simulink library "peripheral_utilities_src"  (R2022b)
settings: Solver=VariableStepAuto  StartTime=0.0  StopTime=10.0  RelTol=1e-3
libraries: $bdroot x16, simulink x5, spsSeriesRLCBranchLib x3, peripheral_utilities x3, spsVoltageMeasurementLib x2, spsMosfetLib x2, spsCurrentMeasurementLib x1, spsSecondOrderFilterLib x1, spsGroundLib x1
(part 2 of 2)

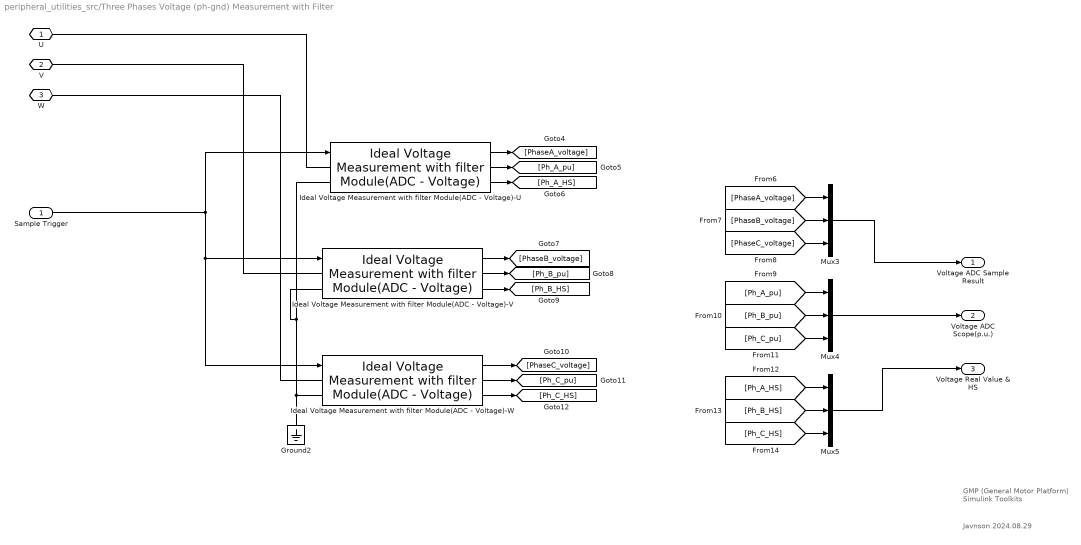
== system peripheral_utilities_src/Three Phases Voltage (ph-gnd) Measurement with Filter ==
  note: Javnson
      | 2024.08.29
  note: GMP (General Motor Platform)
      | Simulink Toolkits
  Sample Trigger : Inport
  Ground2 : spsGroundLib/Ground  LConnTagsString=a
  Ideal Voltage Measurement with filter Module(ADC - Voltage)-U : $bdroot/Ideal Voltage Measurement with filter Module(ADC - Voltage)  ADC_GAIN=ADC_GAIN  ADC_BIT=ADC_BIT  ADC_REFERENCE=ADC_REFERENCE  ADC_BIAS=ADC_BIAS  ADC_INIT=ADC_INIT  cut_frequency=cut_frequency
  Ideal Voltage Measurement with filter Module(ADC - Voltage)-V : $bdroot/Ideal Voltage Measurement with filter Module(ADC - Voltage)  ADC_GAIN=ADC_GAIN  ADC_BIT=ADC_BIT  ADC_REFERENCE=ADC_REFERENCE  ADC_BIAS=ADC_BIAS  ADC_INIT=ADC_INIT  cut_frequency=cut_frequency
  Ideal Voltage Measurement with filter Module(ADC - Voltage)-W : $bdroot/Ideal Voltage Measurement with filter Module(ADC - Voltage)  ADC_GAIN=ADC_GAIN  ADC_BIT=ADC_BIT  ADC_REFERENCE=ADC_REFERENCE  ADC_BIAS=ADC_BIAS  ADC_INIT=ADC_INIT  cut_frequency=cut_frequency
  Mux3 : Mux  Inputs=3
  Mux4 : Mux  Inputs=3
  Mux5 : Mux  Inputs=3
  U : PMIOPort  Side=Left
  V : PMIOPort  Port=2  Side=Left
  W : PMIOPort  Port=3  Side=Left
  Voltage ADC Sample Result : Outport
  Voltage ADC Scope(p.u.) : Outport  Port=2
  Voltage Real Value & HS : Outport  Port=3
  wires:
  Ideal Voltage Measurement with filter Module(ADC - Voltage)-W/3 -> [Ph_C_HS]
  Sample Trigger/1 -> Ideal Voltage Measurement with filter Module(ADC - Voltage)-U/1, Ideal Voltage Measurement with filter Module(ADC - Voltage)-W/1, Ideal Voltage Measurement with filter Module(ADC - Voltage)-V/1
  Ideal Voltage Measurement with filter Module(ADC - Voltage)-V/2 -> [Ph_B_pu]
  Ideal Voltage Measurement with filter Module(ADC - Voltage)-V/3 -> [Ph_B_HS]
  Mux4/1 -> Voltage ADC Scope(p.u.)/1
  [Ph_B_HS] -> Mux5/2
  Ideal Voltage Measurement with filter Module(ADC - Voltage)-W/1 -> [PhaseC_voltage]
  Ideal Voltage Measurement with filter Module(ADC - Voltage)-V/1 -> [PhaseB_voltage]
  Ideal Voltage Measurement with filter Module(ADC - Voltage)-U/1 -> [PhaseA_voltage]
  Ideal Voltage Measurement with filter Module(ADC - Voltage)-U/2 -> [Ph_A_pu]
  [Ph_B_pu] -> Mux4/2
  [PhaseB_voltage] -> Mux3/2
  Ideal Voltage Measurement with filter Module(ADC - Voltage)-U/3 -> [Ph_A_HS]
  Ideal Voltage Measurement with filter Module(ADC - Voltage)-W/2 -> [Ph_C_pu]
  [Ph_A_pu] -> Mux4/1
  [PhaseC_voltage] -> Mux3/3
  [PhaseA_voltage] -> Mux3/1
  [Ph_C_pu] -> Mux4/3
  [Ph_C_HS] -> Mux5/3
  Mux3/1 -> Voltage ADC Sample Result/1
  [Ph_A_HS] -> Mux5/1
  Mux5/1 -> Voltage Real Value & HS/1
  connections:
  Ground2/LConn1 -- Ideal Voltage Measurement with filter Module(ADC - Voltage)-V/LConn2 -- Ideal Voltage Measurement with filter Module(ADC - Voltage)-U/LConn2 -- Ideal Voltage Measurement with filter Module(ADC - Voltage)-W/LConn2
  Ideal Voltage Measurement with filter Module(ADC - Voltage)-U/LConn1 -- U/RConn1
  Ideal Voltage Measurement with filter Module(ADC - Voltage)-V/LConn1 -- V/RConn1
  Ideal Voltage Measurement with filter Module(ADC - Voltage)-W/LConn1 -- W/RConn1

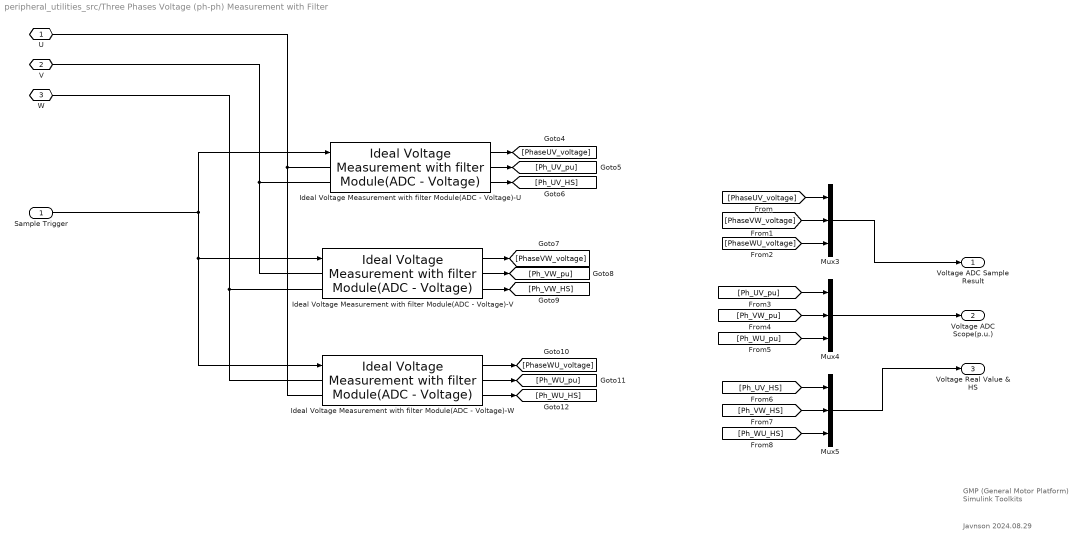
== system peripheral_utilities_src/Three Phases Voltage (ph-ph) Measurement with Filter ==
  note: Javnson
      | 2024.08.29
  note: GMP (General Motor Platform)
      | Simulink Toolkits
  Sample Trigger : Inport
  Ideal Voltage Measurement with filter Module(ADC - Voltage)-U : peripheral_utilities/Ideal Voltage Measurement with filter Module(ADC - Voltage)  ADC_GAIN=ADC_GAIN  ADC_BIT=ADC_BIT  ADC_REFERENCE=ADC_REFERENCE  ADC_BIAS=ADC_BIAS  ADC_INIT=ADC_INIT  cut_frequency=cut_frequency
  Ideal Voltage Measurement with filter Module(ADC - Voltage)-V : peripheral_utilities/Ideal Voltage Measurement with filter Module(ADC - Voltage)  ADC_GAIN=ADC_GAIN  ADC_BIT=ADC_BIT  ADC_REFERENCE=ADC_REFERENCE  ADC_BIAS=ADC_BIAS  ADC_INIT=ADC_INIT  cut_frequency=cut_frequency
  Ideal Voltage Measurement with filter Module(ADC - Voltage)-W : peripheral_utilities/Ideal Voltage Measurement with filter Module(ADC - Voltage)  ADC_GAIN=ADC_GAIN  ADC_BIT=ADC_BIT  ADC_REFERENCE=ADC_REFERENCE  ADC_BIAS=ADC_BIAS  ADC_INIT=ADC_INIT  cut_frequency=cut_frequency
  Mux3 : Mux  Inputs=3
  Mux4 : Mux  Inputs=3
  Mux5 : Mux  Inputs=3
  U : PMIOPort  Side=Left
  V : PMIOPort  Port=2  Side=Left
  W : PMIOPort  Port=3  Side=Left
  Voltage ADC Sample Result : Outport
  Voltage ADC Scope(p.u.) : Outport  Port=2
  Voltage Real Value & HS : Outport  Port=3
  wires:
  Ideal Voltage Measurement with filter Module(ADC - Voltage)-W/3 -> [Ph_WU_HS]
  Sample Trigger/1 -> Ideal Voltage Measurement with filter Module(ADC - Voltage)-U/1, Ideal Voltage Measurement with filter Module(ADC - Voltage)-V/1, Ideal Voltage Measurement with filter Module(ADC - Voltage)-W/1
  Ideal Voltage Measurement with filter Module(ADC - Voltage)-V/2 -> [Ph_VW_pu]
  Ideal Voltage Measurement with filter Module(ADC - Voltage)-V/3 -> [Ph_VW_HS]
  Mux4/1 -> Voltage ADC Scope(p.u.)/1
  [Ph_VW_HS] -> Mux5/2
  Ideal Voltage Measurement with filter Module(ADC - Voltage)-W/1 -> [PhaseWU_voltage]
  Ideal Voltage Measurement with filter Module(ADC - Voltage)-V/1 -> [PhaseVW_voltage]
  Ideal Voltage Measurement with filter Module(ADC - Voltage)-U/1 -> [PhaseUV_voltage]
  Ideal Voltage Measurement with filter Module(ADC - Voltage)-U/2 -> [Ph_UV_pu]
  [Ph_VW_pu] -> Mux4/2
  [PhaseVW_voltage] -> Mux3/2
  Ideal Voltage Measurement with filter Module(ADC - Voltage)-U/3 -> [Ph_UV_HS]
  Ideal Voltage Measurement with filter Module(ADC - Voltage)-W/2 -> [Ph_WU_pu]
  [Ph_UV_pu] -> Mux4/1
  [PhaseWU_voltage] -> Mux3/3
  [PhaseUV_voltage] -> Mux3/1
  [Ph_WU_pu] -> Mux4/3
  [Ph_WU_HS] -> Mux5/3
  Mux3/1 -> Voltage ADC Sample Result/1
  [Ph_UV_HS] -> Mux5/1
  Mux5/1 -> Voltage Real Value & HS/1
  connections:
  Ideal Voltage Measurement with filter Module(ADC - Voltage)-U/LConn1 -- Ideal Voltage Measurement with filter Module(ADC - Voltage)-W/LConn2 -- U/RConn1
  Ideal Voltage Measurement with filter Module(ADC - Voltage)-V/LConn1 -- Ideal Voltage Measurement with filter Module(ADC - Voltage)-U/LConn2 -- V/RConn1
  Ideal Voltage Measurement with filter Module(ADC - Voltage)-W/LConn1 -- Ideal Voltage Measurement with filter Module(ADC - Voltage)-V/LConn2 -- W/RConn1

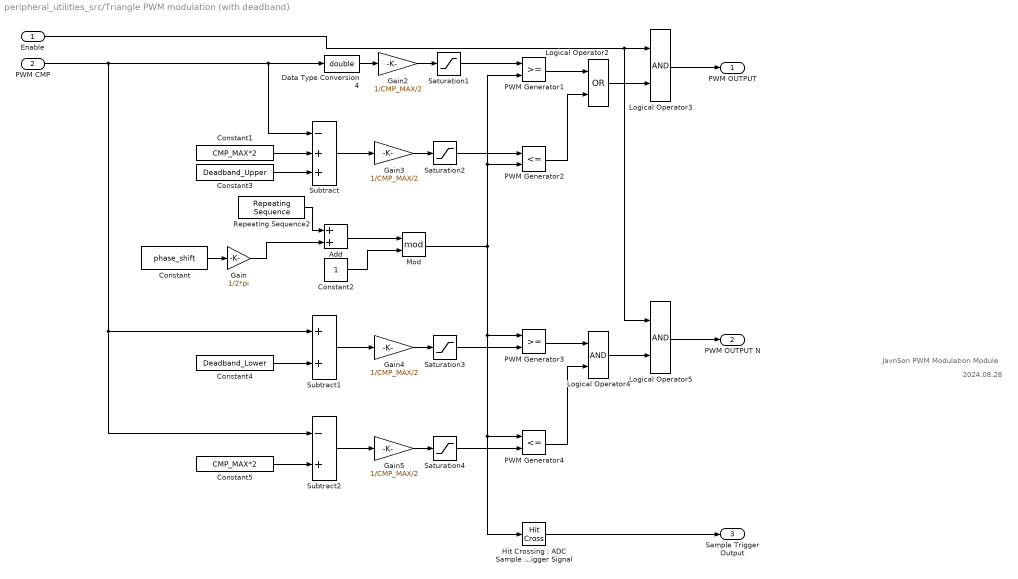
== system peripheral_utilities_src/Triangle PWM modulation (with deadband) ==
  note: 2024.08.28
  note: JavnSon PWM Modulation Module
  Enable : Inport
  PWM CMP : Inport  Port=2
  Add : Sum
  Constant : Constant  Value=phase_shift
  Constant1 : Constant  Value=CMP_MAX*2
  Constant2 : Constant
  Constant3 : Constant  Value=Deadband_Upper
  Constant4 : Constant  Value=Deadband_Lower
  Constant5 : Constant  Value=CMP_MAX*2
  Data Type Conversion4 : DataTypeConversion  OutDataTypeStr=double  SaturateOnIntegerOverflow=off  RndMeth=Floor
  Gain : Gain  Gain=1/2*pi
  Gain{2..5} (4 alike) : Gain  Gain=1/CMP_MAX/2
  Hit Crossing：ADC Sample Trigger Signal : HitCross  HitCrossingOffset=0.5  HitCrossingDirection=rising
  Logical Operator2 : Logic  Operator=OR  AllPortsSameDT=off  OutDataTypeStr=boolean
  Logical Operator3 : Logic  AllPortsSameDT=off  OutDataTypeStr=boolean
  Logical Operator4 : Logic  AllPortsSameDT=off  OutDataTypeStr=boolean
  Logical Operator5 : Logic  AllPortsSameDT=off  OutDataTypeStr=boolean
  Mod : Math  Operator=mod
  PWM Generator1 : RelationalOperator  OutDataTypeStr=boolean  InputSameDT=off
  PWM Generator2 : RelationalOperator  Operator=<=  OutDataTypeStr=boolean  InputSameDT=off
  PWM Generator3 : RelationalOperator  OutDataTypeStr=boolean  InputSameDT=off
  PWM Generator4 : RelationalOperator  Operator=<=  OutDataTypeStr=boolean  InputSameDT=off
  Repeating Sequence2 : simulink/Sources/Repeating Sequence  rep_seq_t=[0, 1/2/fswitch, 1/fswitch ]  rep_seq_y=[0,0.5,1]
  Saturation{1..4} (4 alike) : Saturate  UpperLimit=1  LowerLimit=0
  Subtract : Sum  Inputs=-++
  Subtract1 : Sum
  Subtract2 : Sum  Inputs=-+
  PWM OUTPUT : Outport
  PWM OUTPUT N : Outport  Port=2
  Sample Trigger Output : Outport  Port=3
  wires:
  PWM CMP/1 -> Subtract2/1, Subtract1/1, Subtract/1, Data Type Conversion4/1
  Data Type Conversion4/1 -> Gain2/1
  Gain2/1 -> Saturation1/1
  Saturation1/1 -> PWM Generator1/1
  PWM Generator1/1 -> Logical Operator2/1
  Logical Operator2/1 -> Logical Operator3/2
  Constant1/1 -> Subtract/2
  Constant3/1 -> Subtract/3
  PWM Generator2/1 -> Logical Operator2/2
  Gain3/1 -> Saturation2/1
  Subtract/1 -> Gain3/1
  Saturation2/1 -> PWM Generator2/1
  Constant4/1 -> Subtract1/2
  Gain4/1 -> Saturation3/1
  Subtract1/1 -> Gain4/1
  Saturation3/1 -> PWM Generator3/2
  PWM Generator3/1 -> Logical Operator4/1
  Constant5/1 -> Subtract2/2
  Saturation4/1 -> PWM Generator4/2
  Gain5/1 -> Saturation4/1
  Subtract2/1 -> Gain5/1
  PWM Generator4/1 -> Logical Operator4/2
  Logical Operator4/1 -> Logical Operator5/2
  Mod/1 -> PWM Generator2/2, PWM Generator1/2, PWM Generator3/1, Hit Crossing：ADC Sample Trigger Signal/1, PWM Generator4/1
  Enable/1 -> Logical Operator5/1, Logical Operator3/1
  Logical Operator5/1 -> PWM OUTPUT N/1
  Logical Operator3/1 -> PWM OUTPUT/1
  Hit Crossing：ADC Sample Trigger Signal/1 -> Sample Trigger Output/1
  Repeating Sequence2/1 -> Add/1
  Gain/1 -> Add/2
  Add/1 -> Mod/1
  Constant2/1 -> Mod/2
  Constant/1 -> Gain/1

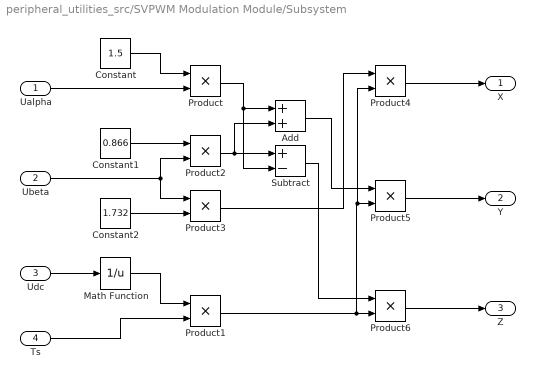
== system peripheral_utilities_src/SVPWM Modulation Module/Subsystem ==
  Ualpha : Inport
  Ubeta : Inport  Port=2
  Udc : Inport  Port=3
  Ts : Inport  Port=4
  Add : Sum
  Constant : Constant  Value=1.5
  Constant1 : Constant  Value=0.866
  Constant2 : Constant  Value=1.732
  Math Function : Math  Operator=reciprocal
  Product{,1..6} (7 alike) : Product
  Subtract : Sum  Inputs=+-
  X : Outport
  Y : Outport  Port=2
  Z : Outport  Port=3
  wires:
  Product1/1 -> Product4/2, Product5/2, Product6/2
  Ts/1 -> Product1/2
  Product6/1 -> Z/1
  Add/1 -> Product5/1
  Ualpha/1 -> Product/2
  Math Function/1 -> Product1/1
  Product2/1 -> Subtract/1, Add/2
  Product4/1 -> X/1
  Product3/1 -> Product4/1
  Constant/1 -> Product/1
  Constant1/1 -> Product2/1
  Ubeta/1 -> Product3/1, Product2/2
  Product5/1 -> Y/1
  Product/1 -> Add/1, Subtract/2
  Constant2/1 -> Product3/2
  Udc/1 -> Math Function/1
  Subtract/1 -> Product6/1

== system peripheral_utilities_src/SVPWM Modulation Module/Subsystem1 ==
  N : Inport
  X : Inport  Port=2
  Y : Inport  Port=3
  Z : Inport  Port=4
  Gain : Gain  Gain=-1
  Gain1 : Gain  Gain=-1
  Gain2 : Gain  Gain=-1
  Multiport Switch : MultiPortSwitch  Inputs=6  DiagnosticForDefault=None  SaturateOnIntegerOverflow=off  InputSameDT=off
  Multiport Switch1 : MultiPortSwitch  Inputs=6  DiagnosticForDefault=None  SaturateOnIntegerOverflow=off  InputSameDT=off
  T1 : Outport
  T2 : Outport  Port=2
  wires:
  Multiport Switch1/1 -> T2/1
  X/1 -> Multiport Switch1/4, Multiport Switch/6, Gain/1
  Y/1 -> Gain1/1, Multiport Switch/3, Multiport Switch1/2
  Z/1 -> Gain2/1, Multiport Switch/2, Multiport Switch1/5
  Gain/1 -> Multiport Switch1/3, Multiport Switch/5
  Gain2/1 -> Multiport Switch/4, Multiport Switch1/7
  N/1 -> Multiport Switch1/1, Multiport Switch/1
  Gain1/1 -> Multiport Switch1/6, Multiport Switch/7
  Multiport Switch/1 -> T1/1

== system peripheral_utilities_src/SVPWM Modulation Module/Subsystem2 ==
  N : Inport
  T1 : Inport  Port=2  Interpolate=off
  T2 : Inport  Port=3
  Ts : Inport  Port=4
  Add : Sum
  Add1 : Sum
  Constant : Constant  Value=0.25
  Constant1 : Constant  Value=0.5
  Constant2 : Constant  Value=0.5
  Multiport Switch : MultiPortSwitch  Inputs=6  DiagnosticForDefault=None  SaturateOnIntegerOverflow=off  InputSameDT=off
  Multiport Switch1 : MultiPortSwitch  Inputs=6  DiagnosticForDefault=None  SaturateOnIntegerOverflow=off  InputSameDT=off
  Multiport Switch2 : MultiPortSwitch  Inputs=6  DiagnosticForDefault=None  SaturateOnIntegerOverflow=off  InputSameDT=off
  Product : Product
  Product1 : Product
  Product2 : Product
  Subtract : Sum  Inputs=--+
  Ta : Outport
  Tb : Outport  Port=2
  Tc : Outport  Port=3
  wires:
  Subtract/1 -> Product/1
  Product1/1 -> Add1/1
  T2/1 -> Product1/1, Subtract/2
  Product/1 -> Add/2, Multiport Switch2/5, Multiport Switch2/7, Multiport Switch/4, Multiport Switch/3, Multiport Switch1/2, Multiport Switch1/6
  Multiport Switch2/1 -> Tc/1
  Add1/1 -> Multiport Switch2/4, Multiport Switch2/2, Multiport Switch1/7, Multiport Switch1/3, Multiport Switch/6, Multiport Switch/5
  N/1 -> Multiport Switch2/1, Multiport Switch1/1, Multiport Switch/1
  Multiport Switch/1 -> Ta/1
  Constant/1 -> Product/2
  Constant2/1 -> Product2/2
  Add/1 -> Add1/2, Multiport Switch1/5, Multiport Switch/7, Multiport Switch/2, Multiport Switch1/4, Multiport Switch2/6, Multiport Switch2/3
  Multiport Switch1/1 -> Tb/1
  Product2/1 -> Add/1
  Constant1/1 -> Product1/2
  T1/1 -> Product2/1, Subtract/1
  Ts/1 -> Subtract/3

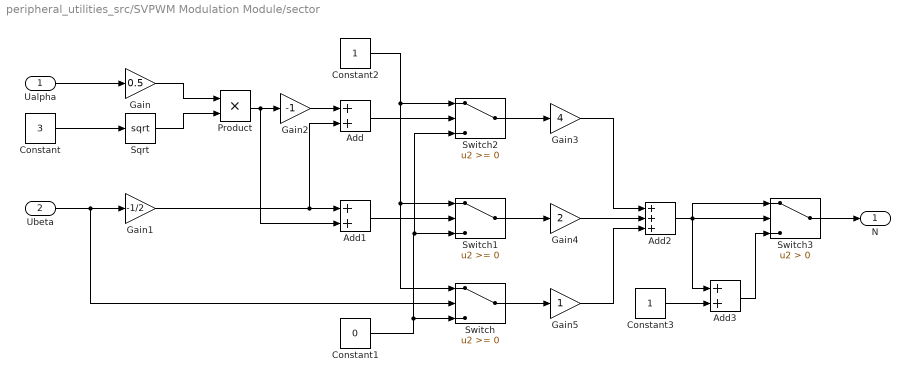
== system peripheral_utilities_src/SVPWM Modulation Module/sector ==
  Ualpha : Inport
  Ubeta : Inport  Port=2
  Add : Sum
  Add1 : Sum
  Add2 : Sum  Inputs=+++
  Add3 : Sum
  Constant : Constant  Value=3
  Constant1 : Constant  Value=0
  Constant2 : Constant
  Constant3 : Constant
  Gain : Gain  Gain=0.5
  Gain1 : Gain  Gain=-1/2
  Gain2 : Gain  Gain=-1
  Gain3 : Gain  Gain=4
  Gain4 : Gain  Gain=2
  Gain5 : Gain
  Product : Product
  Sqrt : Sqrt
  Switch : Switch  SaturateOnIntegerOverflow=off  InputSameDT=off
  Switch1 : Switch  SaturateOnIntegerOverflow=off  InputSameDT=off
  Switch2 : Switch  SaturateOnIntegerOverflow=off  InputSameDT=off
  Switch3 : Switch  Criteria=u2 > Threshold  SaturateOnIntegerOverflow=off  InputSameDT=off
  N : Outport
  wires:
  Gain1/1 -> Add1/1, Add/2
  Constant1/1 -> Switch2/3, Switch1/3, Switch/3
  Gain2/1 -> Add/1
  Gain/1 -> Product/1
  Constant3/1 -> Add3/2
  Add/1 -> Switch2/2
  Product/1 -> Add1/2, Gain2/1
  Sqrt/1 -> Product/2
  Ubeta/1 -> Switch/2, Gain1/1
  Switch/1 -> Gain5/1
  Switch2/1 -> Gain3/1
  Add3/1 -> Switch3/3
  Add2/1 -> Switch3/1, Add3/1, Switch3/2
  Switch3/1 -> N/1
  Gain3/1 -> Add2/1
  Add1/1 -> Switch1/2
  Switch1/1 -> Gain4/1
  Gain4/1 -> Add2/2
  Constant/1 -> Sqrt/1
  Gain5/1 -> Add2/3
  Constant2/1 -> Switch/1, Switch1/1, Switch2/1
  Ualpha/1 -> Gain/1

== matlab function peripheral_utilities_src/SVPWM Module(Ualpha-beta to Tabc, pu)/SVPWM Modulation ==
  data: Ualpha input; T output; Ubeta input; Half_cycle input
function T = fcn(Ualpha, Ubeta, Half_cycle)

T = zeros(3,1);

Ualpha_tmp = -Ualpha/2;
Ubeta_tmp = Ubeta*sqrt(3)/2;

Ua = Ualpha;
Ub = Ualpha_tmp + Ubeta_tmp;
Uc = Ualpha_tmp - Ubeta_tmp;


if (Ua > Ub)
    Umax = Ua;
    Umin = Ub;
else
    Umax = Ub;
    Umin = Ua;
end

if (Uc > Umax)
    Umax = Uc;
elseif (Uc < Umin)
    Umin = Uc;
end

Ucom = (Umax + Umin)/2;

T(1) = Ua - Ucom;
T(2) = Ub - Ucom;
T(3) = Uc - Ucom;

T = (T + 0.5) .* Half_cycle ;
end
